simulink model "suspenstion_of_car"  (R2023a)
settings: Solver=VariableStepAuto  StartTime=0.0  StopTime=10.0  RelTol=1e-3
settings Model: Creator=nayan  LastModifiedBy=nayan

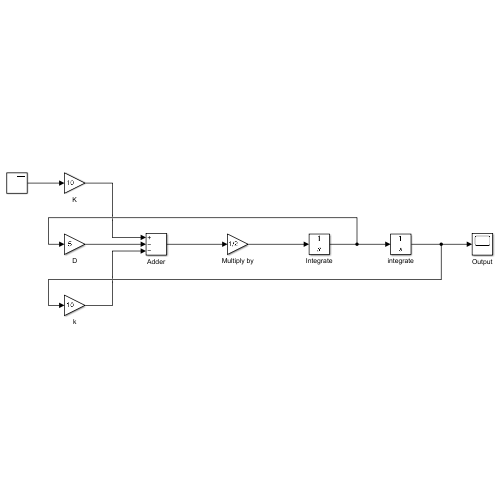
[thumbnail: Simulink's stored preview of the top-level diagram]
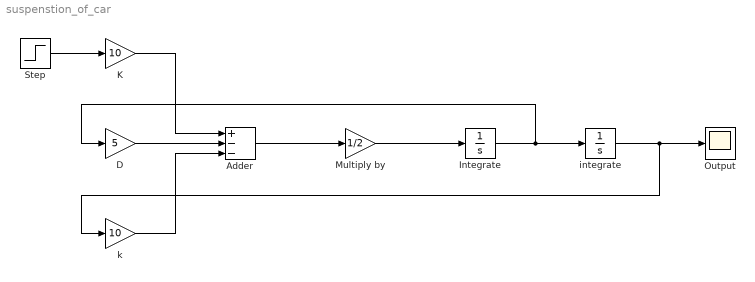
== system suspenstion_of_car ==
  Adder : Sum  Inputs=+--
  D : Gain  Gain=5
  Integrate : Integrator
  K : Gain  Gain=10
  Multiply by : Gain  Gain=1/2
  Output : Scope
  Step : Step  SampleTime=0
  integrate : Integrator
  k : Gain  Gain=10
  wires:
  Adder/1 -> Multiply by/1
  Multiply by/1 -> Integrate/1
  integrate/1 -> k/1, Output/1
  K/1 -> Adder/1
  D/1 -> Adder/2
  k/1 -> Adder/3
  Step/1 -> K/1
  Integrate/1 -> D/1, integrate/1
